simulink model "xyztorgb_fixpt_xsgbbx"  (R2013b)
settings: Solver=FixedStepDiscrete  SolverMode=SingleTasking  StartTime=0.0  StopTime=10.0  RelTol=1e-3
libraries: xbsIndex_r4 x10
settings Model: DataTypeOverride=Off  Creator=Sechw  LastModifiedBy=Sechw
settings DataIOCC: SaveOutput=off  SaveTime=off
settings OptimizationCC: BlockReduction=off  ConditionallyExecuteInputs=off  InlineParams=on
settings DebuggingCC: AlgebraicLoopMsg=error  SingleTaskRateTransMsg=error
settings HardwareCC: ProdHWDeviceType=ASIC/FPGA->ASIC/FPGA  ProdEqTarget=off

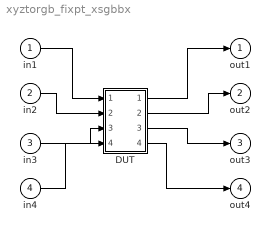
== system xyztorgb_fixpt_xsgbbx ==
  in1 : Inport  OutDataTypeStr=numerictype('boolean')
  in2 : Inport  Port=2  OutDataTypeStr=numerictype(false,8,0)
  in3 : Inport  Port=3  OutDataTypeStr=numerictype(false,8,0)
  in4 : Inport  Port=4  OutDataTypeStr=numerictype(false,8,0)
  DUT : Subsystem
  out1 : Outport
  out2 : Outport  Port=2
  out3 : Outport  Port=3
  out4 : Outport  Port=4
  wires:
  in1/1 -> DUT/1(In1)
  in2/1 -> DUT/2(In2)
  in3/1 -> DUT/3(In3)
  in4/1 -> DUT/4(In4)
  DUT/1(Out1) -> out1/1
  DUT/2(Out2) -> out2/1
  DUT/3(Out3) -> out3/1
  DUT/4(Out4) -> out4/1

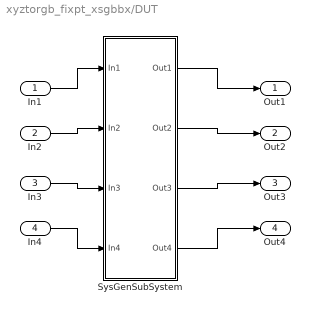
== system xyztorgb_fixpt_xsgbbx/DUT ==
  In1 : Inport
  In2 : Inport  Port=2
  In3 : Inport  Port=3
  In4 : Inport  Port=4
  SysGenSubSystem : Subsystem
  Out1 : Outport
  Out2 : Outport  Port=2
  Out3 : Outport  Port=3
  Out4 : Outport  Port=4
  wires:
  In4/1 -> SysGenSubSystem/4(In4)
  In1/1 -> SysGenSubSystem/1(In1)
  SysGenSubSystem/2(Out2) -> Out2/1
  In2/1 -> SysGenSubSystem/2(In2)
  SysGenSubSystem/1(Out1) -> Out1/1
  In3/1 -> SysGenSubSystem/3(In3)
  SysGenSubSystem/4(Out4) -> Out4/1
  SysGenSubSystem/3(Out3) -> Out3/1

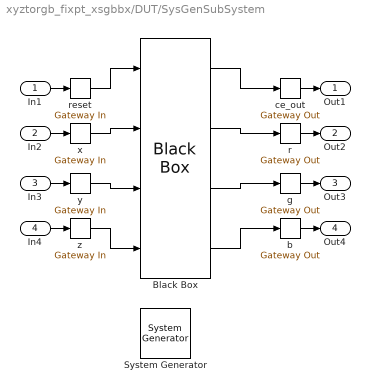
== system xyztorgb_fixpt_xsgbbx/DUT/SysGenSubSystem ==
  In1 : Inport
  In2 : Inport  Port=2
  In3 : Inport  Port=3
  In4 : Inport  Port=4
  " System Generator" : xbsIndex_r4/ System Generator  Tag=genX  xilinxfamily=kintex7  part=xc7k325t  speed=-3  package=fbg676  synthesis_tool=XST  clock_wrapper=Clock Enables  directory=./netlist  proj_type=Project Navigator  Synth_file=XST Defaults  Impl_file=ISE Defaults  testbench=off  simulink_period=1  sysclk_period=10  dcm_input_clock_period=10  incr_netlist=off  trim_vbits=Everywhere in SubSystem  dbl_ovrd=According to Block Masks  core_generation=According to Block Masks  run_coregen=off  deprecated_control=off  eval_field=0  block_type=sysgen
  Black Box : xbsIndex_r4/Black Box  init_code=xyztorgb_fixpt_xsgbbxcfg  sim_method=Inactive  verbose=off  block_type=blackbox2
  b : xbsIndex_r4/Gateway Out  inherit_from_input=on  hdl_port=on  timing_constraint=None  locs_specified=off  LOCs={}  UseAsDAC=off  DACChannel='1'  block_type=gatewayout
  ce_out : xbsIndex_r4/Gateway Out  inherit_from_input=on  hdl_port=on  timing_constraint=None  locs_specified=off  LOCs={}  UseAsDAC=off  DACChannel='1'  block_type=gatewayout
  g : xbsIndex_r4/Gateway Out  inherit_from_input=on  hdl_port=on  timing_constraint=None  locs_specified=off  LOCs={}  UseAsDAC=off  DACChannel='1'  block_type=gatewayout
  r : xbsIndex_r4/Gateway Out  inherit_from_input=on  hdl_port=on  timing_constraint=None  locs_specified=off  LOCs={}  UseAsDAC=off  DACChannel='1'  block_type=gatewayout
  reset : xbsIndex_r4/Gateway In  gui_display_data_type=Fixed-point  arith_type=Boolean  n_bits=16  bin_pt=14  preci_type=Single  exp_width=8  frac_width=24  quantization="Round  (unbiased: +/- Inf)"  overflow=Saturate  period=1  dbl_ovrd=off  timing_constraint=None  locs_specified=off  LOCs={}  UseAsADC=off  ADCChannel='1'  inherit_from_input=off  hdl_port=on  block_type=gatewayin
  x : xbsIndex_r4/Gateway In  gui_display_data_type=Fixed-point  arith_type=Unsigned  n_bits=8  bin_pt=0  preci_type=Single  exp_width=8  frac_width=24  quantization="Round  (unbiased: +/- Inf)"  overflow=Saturate  period=1  dbl_ovrd=off  timing_constraint=None  locs_specified=off  LOCs={}  UseAsADC=off  ADCChannel='1'  inherit_from_input=off  hdl_port=on  block_type=gatewayin
  y : xbsIndex_r4/Gateway In  gui_display_data_type=Fixed-point  arith_type=Unsigned  n_bits=8  bin_pt=0  preci_type=Single  exp_width=8  frac_width=24  quantization="Round  (unbiased: +/- Inf)"  overflow=Saturate  period=1  dbl_ovrd=off  timing_constraint=None  locs_specified=off  LOCs={}  UseAsADC=off  ADCChannel='1'  inherit_from_input=off  hdl_port=on  block_type=gatewayin
  z : xbsIndex_r4/Gateway In  gui_display_data_type=Fixed-point  arith_type=Unsigned  n_bits=8  bin_pt=0  preci_type=Single  exp_width=8  frac_width=24  quantization="Round  (unbiased: +/- Inf)"  overflow=Saturate  period=1  dbl_ovrd=off  timing_constraint=None  locs_specified=off  LOCs={}  UseAsADC=off  ADCChannel='1'  inherit_from_input=off  hdl_port=on  block_type=gatewayin
  Out1 : Outport
  Out2 : Outport  Port=2
  Out3 : Outport  Port=3
  Out4 : Outport  Port=4
  wires:
  b/1 -> Out4/1
  reset/1 -> Black Box/1
  y/1 -> Black Box/3
  x/1 -> Black Box/2
  z/1 -> Black Box/4
  g/1 -> Out3/1
  In4/1 -> z/1
  In1/1 -> reset/1
  r/1 -> Out2/1
  ce_out/1 -> Out1/1
  In3/1 -> y/1
  In2/1 -> x/1
  Black Box/1 -> ce_out/1
  Black Box/2 -> r/1
  Black Box/3 -> g/1
  Black Box/4 -> b/1
